simulink model "part2_3"  (R2018a)
settings: Solver=VariableStepAuto  StartTime=0.0  StopTime=100.0  MaxStep=0.01  RelTol=1e-3
settings Model: Creator=82354  LastModifiedBy=82354

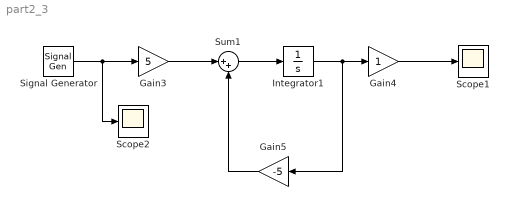
== system part2_3 ==
  Gain3 : Gain  Gain=5
  Gain4 : Gain
  Gain5 : Gain  Gain=-5
  Integrator1 : Integrator
  Scope1 : Scope
  Scope2 : Scope
  Signal Generator : SignalGenerator  Frequency=0.1  Units=rad/sec
  Sum1 : Sum  Inputs=|++
  wires:
  Sum1/1 -> Integrator1/1
  Gain3/1 -> Sum1/1
  Integrator1/1 -> Gain5/1, Gain4/1
  Signal Generator/1 -> Scope2/1, Gain3/1
  Gain5/1 -> Sum1/2
  Gain4/1 -> Scope1/1
